simulink library "can_bus_multi"  (R2018b)
settings: Solver=VariableStepAuto  StartTime=0.0  StopTime=10.0  RelTol=1e-3
libraries: commutil2 x2
settings Model: Creator=Ng Wee Shen  LastModifiedBy=Raymond

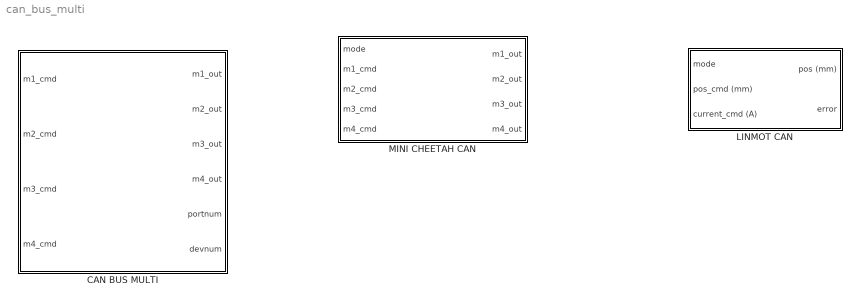
== system can_bus_multi ==
  "CAN BUS MULTI " : Subsystem  TreatAsAtomicUnit=on  SystemSampleTime=PAR_SMPLT  mask(Raspberry Pi CAN Bus){PAR_PORT_NUM=can0, PAR_DEV_NUM=1, PAR_SMPLT=0}
      mask prompts: PAR_PORT_NUM "CAN Port:"; PAR_DEV_NUM "Num. of Device:"; PAR_SMPLT "Sample Time (s):"
      mask help: Raspberry Pi CAN Bus Raspberry Pi CAN Bus Raspberry Pi CAN Bus Raspberry Pi CAN Bus Raspberry Pi CAN Bus Raspberry Pi CAN Bus Raspberry Pi CAN Bus Raspberry Pi CAN Bus
      mask TypeOptions PAR_PORT_NUM: can0 | can1
      mask TypeOptions PAR_DEV_NUM: 1 | 2 | 3 | 4
  LINMOT CAN : Subsystem  TreatAsAtomicUnit=on  SystemSampleTime=PAR_SMPLT  mask(LINMOT CAN (Raspberry Pi)){PAR_MAX_VEL=1, PAR_ACCEL=10, PAR_DECEL=10, PAR_PORT_NUM=can0, PAR_SAFE=on, PAR_SMPLT=0.001}
      mask prompts: PAR_MAX_VEL "Max velocity (m/s)"; PAR_ACCEL "Acceleration (m/s^2)"; PAR_DECEL "Deceleration (m/s^2)"; PAR_PORT_NUM "CAN Port:"; PAR_SAFE "Safe Start"; PAR_SMPLT "Sample Time (s):"
      mask help:
      | Raspberry Pi CAN Bus Driver for LINMOT C1100 Driver.
      |
      | Mode 0: Idle
      | Mode 1: Position control (VAI 16 Bit Go To Pos (090xh))
      | Mode 2: Current control (Current Command Mode (390xh))
      |
      | Configure Position Control parameters, ie: max speed, acceleration and deceleration.
      | Select your CAN port. CAN0 and CAN1 might be flipped.
      |
      | If encounter error, try to fix the problem and then click "Acknowledge error & Reset" to restart. For fatal error, you have to restart the power.
      |
      | Tested on LINMOT SN2 Linear motor, using Raspberry Pi 4B with Waveshare 2-CH CAN HAT, on MATLAB R2018b External mode.
      | 08/4/2021
      mask init:
      | % Get this mask's handle
      | maskObj = Simulink.Mask.get(gcb);
      | 
      | % Get the selected value from mask parameter's option
      | str_PortNum = char(maskObj.Parameters(4).TypeOptions(PAR_PORT_NUM));
      | str_Sample = maskObj.Parameters(6).Value;
      | str_Safe = maskObj.Parameters(5).Value;
      | 
      | 
      | % Set Icon
      | str1 = sprintf('%s',str_PortNum);
      | str2 = sprintf('%ss',str_Sample);
      | 
      | if strcmp(str_Safe,'on')
      |     str3 = sprintf('Safe');
      |     PAR_SAFE = 1;
      | else
      |     str3 = sprintf('');
      |     PAR_SAFE = 0;
      | end
      | 
      | % Set the values of Variant Subsystem
      | str = [str1,'\n',str2,'\n',str3];
      mask Help: https://www.waveshare.com/wiki/2-CH_CAN_HAT
      mask TypeOptions PAR_PORT_NUM: can0 | can1
      mask DialogControl DescTextVar Tooltip: Press 'Help' for more information.
      mask DialogControl Container3 Prompt: Position Cmd Parameters
      mask DialogControl PAR_PORT_NUM Tooltip: can0 and can1 is flipped
      mask DialogControl Control2 Prompt: Acknowledge Error -> Reset
      mask DialogControl Control2 Callback:
      | set_param(gcb+"/PAR_MASK_MODE", 'value', num2str(3));
      | 
      | pause(0.1);
      | 
      | set_param(gcb+"/PAR_MASK_MODE", 'value', num2str(0));
      mask Display: disp(str);
  MINI CHEETAH CAN : Subsystem  TreatAsAtomicUnit=on  SystemSampleTime=PAR_SMPLT  mask(Mini Cheetah CAN (Raspberry Pi)){PAR_PORT_NUM=can1, PAR_SAFE=on, PAR_DEV_NUM=1, PAR_SMPLT=0.001}
      mask prompts: PAR_PORT_NUM "CAN Port:"; PAR_SAFE "Safe Start"; PAR_DEV_NUM "Num. of Device:"; PAR_SMPLT "Sample Time (s):"
      mask help:
      | Rasperry Pi CAN Bus Driver for MIT Mini Cheetah based motor controller.
      | Control up to 4 motors, specify your motors CAN ID in ascending order, ie: 1,2,3,4.
      | CAN Master ID should be 0.
      |
      | -------INPUT-------
      | Connect "mode" to a 1x4 size signal.
      | Mode 0: ExitMotorMode (idle)
      | Mode 1: EnterMotorMode
      |
      | Connect "m#_cmd" to a 1x5 signal of [p v kp kd t_ff], where
      | p: position, v: velocity, kp: p gain, kd: d gain, t_ff: feedforward current
      | Unused "m#_cmd" should be left unconnected.
      |
      | -------OUTPUT-------
      | "m#_out" output a 1x3 size signal of [position, velocity, current] of the motor.
      |
      | -------SET ZERO-------
      | The motor initialize with the zero position configured using UART and can be override with this set zero.
      | This new zero position will NOT be saved to flash memory and will be lost when restart.
      | The zero position configure using UART is saved to the flash memory.
      | Set Zero can be used either in mode 0 or mode 1.
      |
      | -------SAFE START-------
      | All the modes cmd need to be 0 for the first time in order for the motor to operate.
      | Prevent accident when compiling with non zero mode cmd in the start.
      |
      |
      | Tested on T-MOTOR AK80-6, AK60-6, using Raspberry Pi 4B with Waveshare 2-CH CAN HAT, on MATLAB R2018b External mode.
      | 29/3/2021
      mask init:
      | % Get this mask's handle
      | 
      | 
      | maskObj = Simulink.Mask.get(gcb);
      | 
      | % Get the selected value from mask parameter's option
      | str_PortNum = char(maskObj.Parameters(1).TypeOptions(PAR_PORT_NUM));
      | str_DevNum = char(maskObj.Parameters(3).TypeOptions(PAR_DEV_NUM));
      | str_Sample = maskObj.Parameters(4).Value;
      | str_Safe = maskObj.Parameters(2).Value;
      | 
      | 
      | % Set Icon
      | str1 = sprintf('CAN Port: %s',str_PortNum);
      | str2 = sprintf('Number of Device: %s',str_DevNum);
      | str3 = sprintf('Sample Time: %ss',str_Sample);
      | 
      | 
      | 
      | if strcmp(str_Safe,'on')
      |     str4 = sprintf('Safe');
      |     PAR_SAFE = 1;
      | else
      |     str4 = sprintf('');
      |     PAR_SAFE = 0;
      | end
      | 
      | 
      | % Set the values of Variant Subsystem
      | str = [str1,'\n',str2,'\n',str3,'\n',str4];
      settings: MinAlgLoopOccurrences=on
      mask Help:
      | https://www.waveshare.com/wiki/2-CH_CAN_HAT
      | https://os.mbed.com/users/benkatz/code/HKC_MiniCheetah/
      | https://os.mbed.com/users/benkatz/code/SPIne/
      mask TypeOptions PAR_PORT_NUM: can0 | can1
      mask TypeOptions PAR_DEV_NUM: 1 | 2 | 3 | 4
      mask Callback PAR_DEV_NUM:
      | p = Simulink.Mask.get(gcb);
      | 
      | ctrl2 = p.getDialogControl("Control2");
      | ctrl3 = p.getDialogControl("Control3");
      | ctrl4 = p.getDialogControl("Control4");
      | ctrl5 = p.getDialogControl("Control5");
      | 
      | switch get_param(gcb,'PAR_DEV_NUM')
      |     case '1'
      |         ctrl2.Enabled = 'on';
      |         ctrl3.Enabled = 'off';
      |         ctrl4.Enabled = 'off';
      |         ctrl5.Enabled = 'off';
      |     case '2'
      |         ctrl2.Enabled = 'on';
      |         ctrl3.Enabled = 'on';
      |         ctrl4.Enabled = 'off';
      |         ctrl5.Enabled = 'off';
      |     case '3'
      |         ctrl2.Enabled = 'on';
      |         ctrl3.Enabled = 'on';
      |         ctrl4.Enabled = 'on';
      |         ctrl5.Enabled = 'off';
      |     case '4'
      |         ctrl2.Enabled = 'on';
      |         ctrl3.Enabled = 'on';
      |         ctrl4.Enabled = 'on';
      |         ctrl5.Enabled = 'on';
      | end
      mask DialogControl DescTextVar Tooltip: Press 'Help' for more information.
      mask DialogControl Container3 Prompt: Set Zero
      mask DialogControl Control2 Prompt: Motor 1
      mask DialogControl Control2 Callback:
      | set_param(gcb+"/PAR_MASK_MODE", 'value', mat2str([2 0 0 0]));
      | 
      | pause(0.1);
      | 
      | set_param(gcb+"/PAR_MASK_MODE", 'value', mat2str([0 0 0 0]));
      mask DialogControl Control3 Prompt: Motor 2
      mask DialogControl Control3 Callback:
      | set_param(gcb+"/PAR_MASK_MODE", 'value', mat2str([0 2 0 0]));
      | 
      | pause(0.1);
      | 
      | set_param(gcb+"/PAR_MASK_MODE", 'value', mat2str([0 0 0 0]));
      mask DialogControl Control4 Prompt: Motor 3
      mask DialogControl Control4 Callback:
      | set_param(gcb+"/PAR_MASK_MODE", 'value', mat2str([0 0 2 0]));
      | 
      | pause(0.1);
      | 
      | set_param(gcb+"/PAR_MASK_MODE", 'value', mat2str([0 0 0 0]));
      mask DialogControl Control5 Prompt: Motor 4
      mask DialogControl Control5 Callback:
      | set_param(gcb+"/PAR_MASK_MODE", 'value', mat2str([0 0 0 2]));
      | 
      | pause(0.1);
      | 
      | set_param(gcb+"/PAR_MASK_MODE", 'value', mat2str([0 0 0 0]));
      mask Display: disp(str)

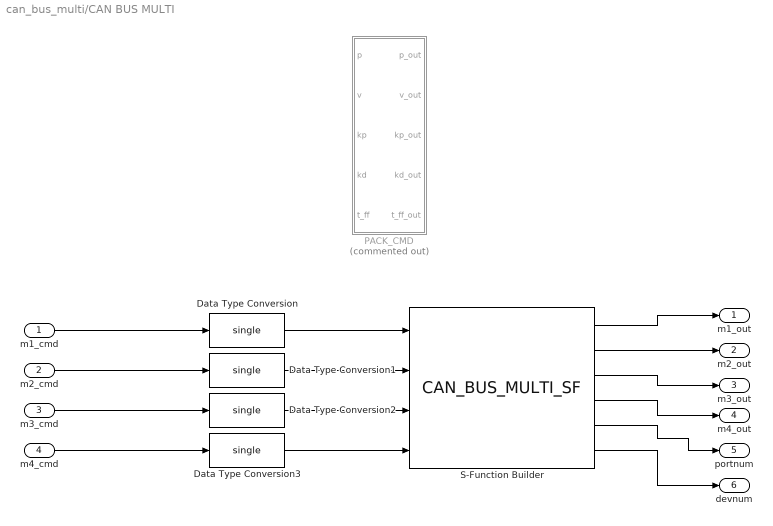
== system can_bus_multi/CAN BUS MULTI  ==
  m1_cmd : Inport
  m2_cmd : Inport  Port=2
  m3_cmd : Inport  Port=3
  m4_cmd : Inport  Port=4
  Data Type Conversion{,1..3} (4 alike) : DataTypeConversion  OutDataTypeStr=single
  PACK_CMD : MATLAB Function  Commented=on  TreatAsAtomicUnit=on
  S-Function Builder : S-Function  InitFcn=try, set_param(gcb,'FunctionName','CAN_BUS_MULTI_SF'), end  FunctionName=CAN_BUS_MULTI_SF  Parameters=uint8(PAR_DEV_NUM),uint8(PAR_PORT_NUM)  SFunctionModules=CAN_BUS_MULTI_SF_wrapper  SFunctionDeploymentMode=off  EnableBusSupport=off  mask(S-Function Builder){}
      mask help: Simulink:masks:SFunctionBuilder_MD
      mask init:
      | val = [[.9  0.75 0.75 1 1 .9 .9 1]',[1 1 0.75 0.75 .9 .9 1 .9]'];try , sys = get_param(gcb,'SfunBuilderFcnName');if isempty(sys), sys = get_param(gcb,'FunctionName'); end,catch, sys = get_param(gcb,'FunctionName'); end
      settings: CopyFcn=set_param(gcbh,'LinkStatus','none')  PreSaveFcn=try, set_param(gcb,'FunctionName','CAN_BUS_MULTI_SF'), end  OpenFcn=sfunctionwizard(gcbh)
      mask Display: plot(val(:,1),val(:,2)),disp(sys), port_label('input',1,'m1_cmd'), port_label('input',2,'m2_cmd'), port_label('input',3,'m3_cmd'), port_label('input',4,'m4_cmd'), port_label('output',1,'m1_out'), port_label('output',2,'m2_out'), port_label('output',3,'m3_out'), port_label('output',4,'m4_out'), port_label('output',5,'err_no'), port_label('output',6,'device_err')
  m1_out : Outport
  m2_out : Outport  Port=2
  m3_out : Outport  Port=3
  m4_out : Outport  Port=4
  portnum : Outport  Port=5
  devnum : Outport  Port=6
  wires:
  S-Function Builder/1 -> m1_out/1
  m1_cmd/1 -> Data Type Conversion/1
  Data Type Conversion/1 -> S-Function Builder/1
  Data Type Conversion1/1 -> S-Function Builder/2
  m2_cmd/1 -> Data Type Conversion1/1
  m4_cmd/1 -> Data Type Conversion3/1
  Data Type Conversion2/1 -> S-Function Builder/3
  Data Type Conversion3/1 -> S-Function Builder/4
  m3_cmd/1 -> Data Type Conversion2/1
  S-Function Builder/6 -> devnum/1
  S-Function Builder/5 -> portnum/1
  S-Function Builder/2 -> m2_out/1
  S-Function Builder/3 -> m3_out/1
  S-Function Builder/4 -> m4_out/1

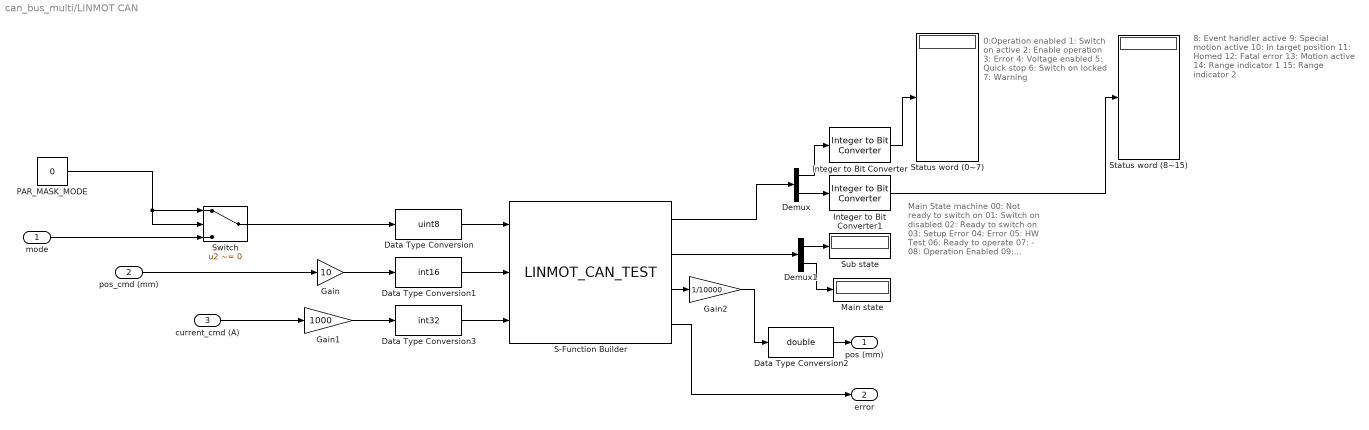
== system can_bus_multi/LINMOT CAN ==
  note: 0:Operation enabled
      | 1: Switch on active
      | 2: Enable operation
      | 3: Error
      | 4: Voltage enabled
      | 5: Quick stop
      | 6: Switch on locked
      | 7: Warning
  note: 8: Event handler active
      | 9: Special motion active
      | 10: In target position
      | 11: Homed
      | 12: Fatal error
      | 13: Motion active
      | 14: Range indicator 1
      | 15: Range indicator 2
  note: Main State machine
      | 00: Not ready to switch on
      | 01: Switch on disabled
      | 02: Ready to switch on
      | 03: Setup Error
      | 04: Error
      | 05: HW Test
      | 06: Ready to operate
      | 07: -
      | 08: Operation Enabled
      | 09: Homing
      | 10: Clearance check
      | 11: Going to initial position
      | 12: Aborting
      | 13: Freezing
      | 14: Quick stop
      | 15: Going to position
      | 16: Jogging+
      | 17: Jogging-
      | 18: Linearizing
      | 19: Phase search
      | 20: Special mode
      | 21: Brake delay
  mode : Inport
  pos_cmd (mm) : Inport  Port=2
  current_cmd (A) : Inport  Port=3
  Data Type Conversion : DataTypeConversion  OutDataTypeStr=uint8
  Data Type Conversion1 : DataTypeConversion  OutDataTypeStr=int16
  Data Type Conversion2 : DataTypeConversion  OutDataTypeStr=double
  Data Type Conversion3 : DataTypeConversion  OutDataTypeStr=int32
  Demux : Demux  Outputs=2
  Demux1 : Demux  Outputs=2
  Gain : Gain  Gain=10
  Gain1 : Gain  Gain=1000
  Gain2 : Gain  Gain=1/10000
  Integer to Bit Converter : commutil2/Integer to Bit Converter  nbits=8  signedInputValues=Unsigned  bitOrder=LSB first  outDtype=Inherit via internal rule
  Integer to Bit Converter1 : commutil2/Integer to Bit Converter  nbits=8  signedInputValues=Unsigned  bitOrder=LSB first  outDtype=Inherit via internal rule
  Main state : Display
  PAR_MASK_MODE : Constant  Value=0  SampleTime=-1
  S-Function Builder : S-Function  InitFcn=try, set_param(gcb,'FunctionName','LINMOT_CAN_TEST'), end  FunctionName=LINMOT_CAN_TEST  Parameters=uint8(PAR_PORT_NUM),PAR_MAX_VEL,PAR_ACCEL,PAR_DECEL,uint8(PAR_SAFE)  SFunctionModules=LINMOT_CAN_TEST_wrapper  SFunctionDeploymentMode=off  EnableBusSupport=off  mask(S-Function Builder){}
      mask help: Simulink:masks:SFunctionBuilder_MD
      mask init: same as can_bus_multi/CAN BUS MULTI /S-Function Builder
      settings: CopyFcn=set_param(gcbh,'LinkStatus','none')  PreSaveFcn=try, set_param(gcb,'FunctionName','LINMOT_CAN_TEST'), end  OpenFcn=sfunctionwizard(gcbh)
      mask Display: plot(val(:,1),val(:,2)),disp(sys), port_label('input',1,'mode'), port_label('input',2,'pos_cmd'), port_label('input',3,'current_cmd'), port_label('output',1,'status_word'), port_label('output',2,'state_var'), port_label('output',3,'position'), port_label('output',4,'err_no')
  Status word (0~7) : Display
  Status word (8~15) : Display
  Sub state : Display
  Switch : Switch  Criteria=u2 ~= 0
      settings: LockScale=on
  pos (mm) : Outport
  error : Outport  Port=2
  wires:
  S-Function Builder/1 -> Demux/1
  Switch/1 -> Data Type Conversion/1
  pos_cmd (mm)/1 -> Gain/1
  Gain1/1 -> Data Type Conversion3/1
  current_cmd (A)/1 -> Gain1/1
  Data Type Conversion3/1 -> S-Function Builder/3
  Gain/1 -> Data Type Conversion1/1
  Demux/1 -> Integer to Bit Converter/1
  Integer to Bit Converter/1 -> Status word (0~7)/1
  Demux/2 -> Integer to Bit Converter1/1
  Integer to Bit Converter1/1 -> Status word (8~15)/1
  Demux1/1 -> Sub state/1
  S-Function Builder/2 -> Demux1/1
  Demux1/2 -> Main state/1
  Gain2/1 -> Data Type Conversion2/1
  S-Function Builder/4 -> error/1
  S-Function Builder/3 -> Gain2/1
  PAR_MASK_MODE/1 -> Switch/2, Switch/1
  mode/1 -> Switch/3
  Data Type Conversion/1 -> S-Function Builder/1
  Data Type Conversion1/1 -> S-Function Builder/2
  Data Type Conversion2/1 -> pos (mm)/1

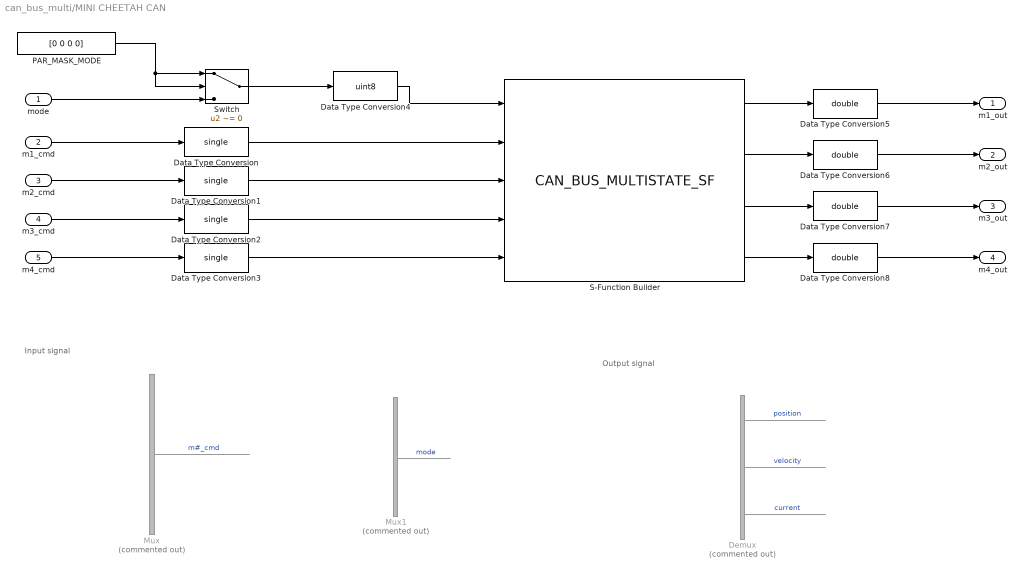
== system can_bus_multi/MINI CHEETAH CAN ==
  note: Input signal
  note: Output signal
  mode : Inport
  m1_cmd : Inport  Port=2
  m2_cmd : Inport  Port=3
  m3_cmd : Inport  Port=4
  m4_cmd : Inport  Port=5
  Data Type Conversion{,1..3} (4 alike) : DataTypeConversion  OutDataTypeStr=single
  Data Type Conversion4 : DataTypeConversion  OutDataTypeStr=uint8
  Data Type Conversion{5..8} (4 alike) : DataTypeConversion  OutDataTypeStr=double
  Demux : Demux  Commented=on  Outputs=3
  Mux : Mux  Commented=on  Inputs=5
  Mux1 : Mux  Commented=on
  PAR_MASK_MODE : Constant  Value=[0 0 0 0]
  S-Function Builder : S-Function  InitFcn=try, set_param(gcb,'FunctionName','CAN_BUS_MULTISTATE_SF'), end  FunctionName=CAN_BUS_MULTISTATE_SF  Parameters=uint8(PAR_DEV_NUM),uint8(PAR_PORT_NUM),uint8(PAR_SAFE)  SFunctionModules=CAN_BUS_MULTISTATE_SF_wrapper  SFunctionDeploymentMode=off  EnableBusSupport=off  mask(S-Function Builder){}
      mask help: Simulink:masks:SFunctionBuilder_MD
      mask init: same as can_bus_multi/CAN BUS MULTI /S-Function Builder
      settings: CopyFcn=set_param(gcbh,'LinkStatus','none')  PreSaveFcn=try, set_param(gcb,'FunctionName','CAN_BUS_MULTISTATE_SF'), end  OpenFcn=sfunctionwizard(gcbh)
      mask Display: plot(val(:,1),val(:,2)),disp(sys), port_label('input',1,'mode'), port_label('input',2,'m1_cmd'), port_label('input',3,'m2_cmd'), port_label('input',4,'m3_cmd'), port_label('input',5,'m4_cmd'), port_label('output',1,'m1_out'), port_label('output',2,'m2_out'), port_label('output',3,'m3_out'), port_label('output',4,'m4_out')
  Switch : Switch  Criteria=u2 ~= 0
  m1_out : Outport
  m2_out : Outport  Port=2
  m3_out : Outport  Port=3
  m4_out : Outport  Port=4
  wires:
  S-Function Builder/3 -> Data Type Conversion7/1
  m1_cmd/1 -> Data Type Conversion/1
  m4_cmd/1 -> Data Type Conversion3/1
  S-Function Builder/2 -> Data Type Conversion6/1
  m3_cmd/1 -> Data Type Conversion2/1
  S-Function Builder/1 -> Data Type Conversion5/1
  m2_cmd/1 -> Data Type Conversion1/1
  S-Function Builder/4 -> Data Type Conversion8/1
  Data Type Conversion4/1 -> S-Function Builder/1
  PAR_MASK_MODE/1 -> Switch/2, Switch/1
  mode/1 -> Switch/3
  Switch/1 -> Data Type Conversion4/1
  Data Type Conversion/1 -> S-Function Builder/2
  Data Type Conversion1/1 -> S-Function Builder/3
  Data Type Conversion2/1 -> S-Function Builder/4
  Data Type Conversion3/1 -> S-Function Builder/5
  Mux/1 -> ?  "m#_cmd"
  ? -> Mux/1  "desired position"
  ? -> Mux/2  "desired velocity"
  ? -> Mux/3  "kp"
  ? -> Mux/4  "kd"
  ? -> Mux/5  "feedforward current"
  ? -> Demux/1  "m#_out"
  Demux/1 -> ?  "position"
  Demux/2 -> ?  "velocity"
  Demux/3 -> ?  "current"
  Mux1/1 -> ?  "mode"
  ? -> Mux1/1  "m1 mode"
  ? -> Mux1/2  "m2 mode"
  ? -> Mux1/3  "m3 mode"
  ? -> Mux1/4  "m4 mode"
  Data Type Conversion5/1 -> m1_out/1
  Data Type Conversion6/1 -> m2_out/1
  Data Type Conversion7/1 -> m3_out/1
  Data Type Conversion8/1 -> m4_out/1

== matlab function can_bus_multi/CAN BUS MULTI /PACK_CMD ==
  data: p input; p_out output; v input; kp input; kd input; t_ff input; v_out output; kp_out output; kd_out output; t_ff_out output
function [p_out, v_out, kp_out, kd_out, t_ff_out] = fcn(p, v, kp, kd, t_ff)



p_out = uint16((p-(-12.5)) * (bitshift(1,16)-1)/(12.5-(-12.5)));

v_out = uint16((v-(-65.0)) * (bitshift(1,12)-1)/(65.0-(-65.0)));

kp_out = uint16((kp-(0.0)) * (bitshift(1,12)-1)/(500.0-(0.0)));

kd_out = uint16((kd-(0.0)) * (bitshift(1,12)-1)/(5.0-(0.0)));

t_ff_out = uint16((t_ff-(-18.0)) * (bitshift(1,12)-1)/(18.0-(-18.0)));
